simulink model "BLAC1_BLOCKS"  (R2018b)
settings: Solver=VariableStepAuto  StartTime=0.0  StopTime=10.0  RelTol=1e-3
settings Model: Creator=anton  LastModifiedBy=anton

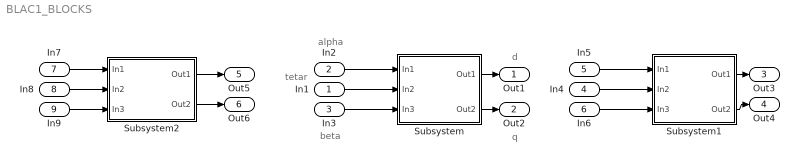
== system BLAC1_BLOCKS ==
  note: q
  note: d
  note: tetar
  note: beta
  note: alpha
  In1 : Inport
  In2 : Inport  Port=2
  In3 : Inport  Port=3
  In4 : Inport  Port=4
  In5 : Inport  Port=5
  In6 : Inport  Port=6
  In7 : Inport  Port=7
  In8 : Inport  Port=8
  In9 : Inport  Port=9
  Subsystem : Subsystem
      mask Display: disp('alfa-beta--->d-q')
  Subsystem1 : Subsystem
      mask Display: disp('d-q--->alfa-beta')
  Subsystem2 : Subsystem
      mask Display: disp('a-b-c--->alfa-beta')
  Out1 : Outport
  Out2 : Outport  Port=2
  Out3 : Outport  Port=3
  Out4 : Outport  Port=4
  Out5 : Outport  Port=5
  Out6 : Outport  Port=6
  wires:
  In2/1 -> Subsystem/1(In1)
  In1/1 -> Subsystem/2(In2)
  In3/1 -> Subsystem/3(In3)
  Subsystem/1(Out1) -> Out1/1
  Subsystem/2(Out2) -> Out2/1
  In5/1 -> Subsystem1/1(In1)
  In4/1 -> Subsystem1/2(In2)
  In6/1 -> Subsystem1/3(In3)
  Subsystem1/1(Out1) -> Out3/1
  Subsystem1/2(Out2) -> Out4/1
  In7/1 -> Subsystem2/1(In1)
  In8/1 -> Subsystem2/2(In2)
  In9/1 -> Subsystem2/3(In3)
  Subsystem2/1(Out1) -> Out5/1
  Subsystem2/2(Out2) -> Out6/1

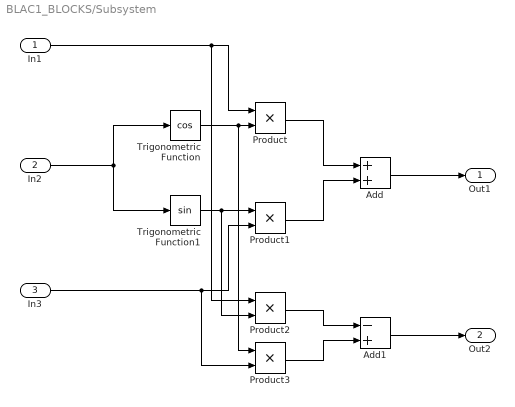
== system BLAC1_BLOCKS/Subsystem ==
  In1 : Inport
  In2 : Inport  Port=2
  In3 : Inport  Port=3
  Add : Sum
  Add1 : Sum  Inputs=-+
  Product{,1..3} (4 alike) : Product
  Trigonometric Function : Trigonometry  Operator=cos
  Trigonometric Function1 : Trigonometry
  Out1 : Outport
  Out2 : Outport  Port=2
  wires:
  Trigonometric Function1/1 -> Product2/2, Product1/1
  Trigonometric Function/1 -> Product3/1, Product/2
  In1/1 -> Product2/1, Product/1
  Product1/1 -> Add/2
  Product2/1 -> Add1/1
  Add1/1 -> Out2/1
  Product3/1 -> Add1/2
  In3/1 -> Product3/2, Product1/2
  Product/1 -> Add/1
  In2/1 -> Trigonometric Function1/1, Trigonometric Function/1
  Add/1 -> Out1/1

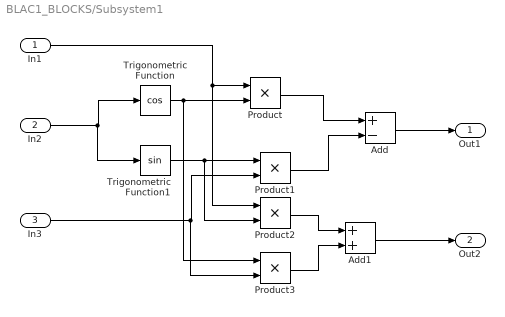
== system BLAC1_BLOCKS/Subsystem1 ==
  In1 : Inport
  In2 : Inport  Port=2
  In3 : Inport  Port=3
  Add : Sum  Inputs=+-
  Add1 : Sum
  Product{,1..3} (4 alike) : Product
  Trigonometric Function : Trigonometry  Operator=cos
  Trigonometric Function1 : Trigonometry
  Out1 : Outport
  Out2 : Outport  Port=2
  wires:
  Trigonometric Function1/1 -> Product2/2, Product1/1
  In1/1 -> Product2/1, Product/1
  Product1/1 -> Add/2
  Product2/1 -> Add1/1
  Product3/1 -> Add1/2
  Product/1 -> Add/1
  In2/1 -> Trigonometric Function1/1, Trigonometric Function/1
  Trigonometric Function/1 -> Product3/1, Product/2
  In3/1 -> Product3/2, Product1/2
  Add1/1 -> Out2/1
  Add/1 -> Out1/1

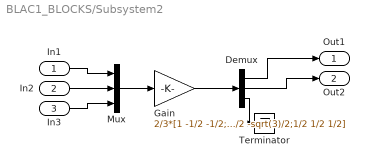
== system BLAC1_BLOCKS/Subsystem2 ==
  In1 : Inport
  In2 : Inport  Port=2
  In3 : Inport  Port=3
  Demux : Demux  Outputs=3
  Gain : Gain  Gain=2/3*[1 -1/2 -1/2;0 sqrt(3)/2 -sqrt(3)/2;1/2 1/2 1/2]
  Mux : Mux  Inputs=3
  Terminator : Terminator
  Out1 : Outport
  Out2 : Outport  Port=2
  wires:
  In2/1 -> Mux/2
  Demux/3 -> Terminator/1
  Demux/2 -> Out2/1
  Mux/1 -> Gain/1
  Demux/1 -> Out1/1
  In3/1 -> Mux/3
  Gain/1 -> Demux/1
  In1/1 -> Mux/1
